simulink model "lttleloopwithLofVenogopal"  (R2017a)
settings: Solver=ode4  StartTime=0.0  StopTime=10  FixedStep=0.0001  RelTol=1e-3
settings Model: Creator=sganzel  LastModifiedBy=sganzel

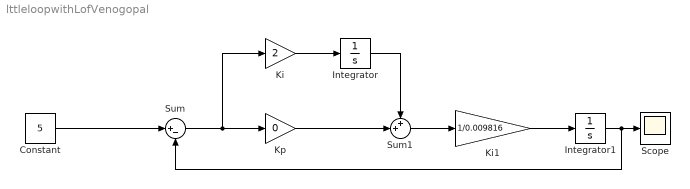
== system lttleloopwithLofVenogopal ==
  Constant : Constant  Value=5
  Integrator : Integrator
  Integrator1 : Integrator
  Ki : Gain  Gain=2
  Ki1 : Gain  Gain=1/0.009816
  Kp : Gain  Gain=0
  Scope : Scope
  Sum : Sum  Inputs=|+-
  Sum1 : Sum  Inputs=++|
  wires:
  Constant/1 -> Sum/1
  Sum/1 -> Ki/1, Kp/1
  Kp/1 -> Sum1/2
  Ki/1 -> Integrator/1
  Integrator/1 -> Sum1/1
  Sum1/1 -> Ki1/1
  Integrator1/1 -> Scope/1, Sum/2
  Ki1/1 -> Integrator1/1
